simulink model "KITTRacing"  (R2016b)
settings: Solver=VariableStepAuto  StartTime=0.0  StopTime=5  MaxStep=0.01  RelTol=1e-3
values from neighbouring files (symbols this model uses):
  b = 0.0015    [KITTParameters.m]
  c = 0.02    [KITTParameters.m]
  F_a = 0    [KITTDriver.m]
  F_b = F_b_max    [KITTDriver.m]
  m = 13    [KITTParameters.m]
  v_0 = 12    [KITTDriver.m]
settings Model: Creator=sumeetsharma  LastModifiedBy=Sieger

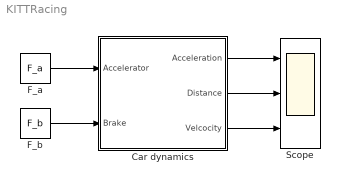
== system KITTRacing ==
  Car dynamics : Subsystem
  F_a : Constant  Value=F_a
  "F_b " : Constant  Value=F_b
  Scope : Scope  NumInputPorts=3
  wires:
  F_a/1 -> Car dynamics/1(Accelerator)
  "F_b "/1 -> Car dynamics/2(Brake)
  Car dynamics/1(Acceleration) -> Scope/1
  Car dynamics/2(Distance) -> Scope/2
  Car dynamics/3(Velcocity) -> Scope/3

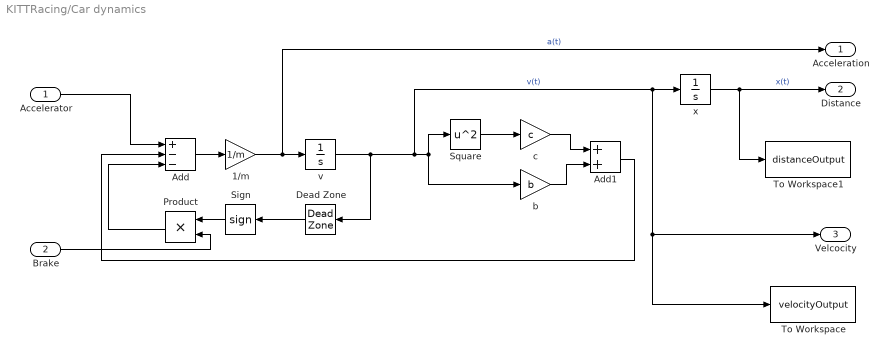
== system KITTRacing/Car dynamics ==
  Accelerator : Inport
  Brake : Inport  Port=2
  1/m : Gain  Gain=1/m
  Add : Sum  Inputs=+--
  Add1 : Sum
  Dead Zone : DeadZone  LowerValue=-0.001  UpperValue=0.001  SaturateOnIntegerOverflow=on
  Product : Product
  Sign : Signum
  Square : Math  Operator=square  SaturateOnIntegerOverflow=on
  To Workspace : ToWorkspace  VariableName=velocityOutput  SaveFormat=Structure With Time  SampleTime=-1
  To Workspace1 : ToWorkspace  VariableName=distanceOutput  SaveFormat=Structure With Time  SampleTime=-1
  b : Gain  Gain=b
  c : Gain  InitFcn=run KITTParameters.m  Gain=c
  v : Integrator  InitialCondition=v_0
  "x " : Integrator
  Acceleration : Outport
  Distance : Outport  Port=2
  Velcocity : Outport  Port=3
  wires:
  Square/1 -> c/1
  Accelerator/1 -> Add/1
  Add/1 -> 1/m/1
  c/1 -> Add1/1
  b/1 -> Add1/2
  1/m/1 -> Acceleration/1, v/1  "a(t)"
  "x "/1 -> To Workspace1/1, Distance/1  "x(t)"
  v/1 -> Dead Zone/1, Velcocity/1, To Workspace/1, "x "/1, b/1, Square/1  "v(t)"
  Add1/1 -> Add/2
  Sign/1 -> Product/1
  Product/1 -> Add/3
  Dead Zone/1 -> Sign/1
  Brake/1 -> Product/2
